simulink model "IEEE68_BUS"  (R2019b)
settings: Solver=ode15s  StartTime=0.0  StopTime=10.0  FixedStep=Ts  RelTol=1e-3
PreLoadFcn:
  | Ts=50e-5;
  | 
  | % Required data to 68 Bus benchmark
  | % clear
  | % clc
  | % Definition for the columns
  | % system base =100 MVA
  | 
  | %% Line data Format (line)
  | % All values are given on the same system base MVA
  | % 1: From bus
  | % 2: To bus
  | % 3: Resistance (pu)
  | % 4: Reactance  (pu)
  | % 5: Charge     (pu)
  | % 6: Transformer Tap Amplitute
  | % 7: base MVA
  | % 8: Nomonal Voltage (KV)
  | 
  | %1   2    3        4       5       6        7      8
  | line=[...
  | 1	54	0	     0.0181	  0	      1.025     100    138
  | 2	58	0	     0.025	  0	      1.070     100    138
  | 3	62	0	     0.02	  0	      1.070     100    138
  | 4	19	0.0007	 0.0142	  0	      1.070     100    138
  | 5	20	0.0009	 0.018	  0	      1.009     100    138
  | 6	22	0	     0.0143	  0	      1.025     100    138
  | 7	23	0.0005	 0.0272	  0	      0         100    138
  | 8	25	0.0006	 0.0232	  0	      1.025     100    138
  | 9	29	0.0008	 0.0156   0	      1.025     100    138
  | 10	31	0	     0.026	  0	      1.04      100    138
  | 11	32	0	     0.013	  0	      1.04      100    138
  | 12	36	0	     0.0075	  0	      1.04      100    138
  | 13	17	0	     0.0033	  0	      1.04      100    138
  | 14	41	0	     0.0015	  0	      1         100    138
  | 15	42	0	     0.0015	  0	      1         100    138
  | 16	18	0	     0.003	  0	      1         100    138
  | 17	36	0.0005	 0.0045	  0.32	  0         100    138
  | 17	43	0.0005	 0.0276	  0	      0         100    138
  | 18	42	0.004	 0.06	  2.25    0         100    138
  | 18	49	0.0076	 0.1141	  1.16    0	        100    138
  | 18	50	0.0012	 0.0288	  2.06	  0         100    138
  | 20	19	0.0007	 0.0138	  0       1.06	    100    138
  | 19	68	0.0016	 0.0195	  0.304	  0         100    138
  | 21	22	0.0008	 0.014	  0.2565  0	        100    138
  | 21	68	0.0008	 0.0135	  0.2548  0	        100    138
  | 22	23	0.0006	 0.0096	  0.1846  0	        100    138
  | 23	24	0.0022	 0.035	  0.361	  0         100    138
  | 24	68	0.0003	 0.0059	  0.068	  0         100    138
  | 25	26	0.0032	 0.0323	  0.531	  0         100    138
  | 25	54	0.007	 0.0086	  0.146	  0         100    138
  | 26	27	0.0014	 0.0147	  0.2396  0	        100    138
  | 26	28	0.0043	 0.0474	  0.7802  0	        100    138
  | 26	29	0.0057	 0.0625	  1.029	  0         100    138
  | 27	37	0.0013	 0.0173	  0.3216  0	        100    138
  | 27	53	0.032	 0.32	  0.41	  0         100    138
  | 29	28	0.0014	 0.0151	  0.249	  0         100    138
  | 30	31	0.0013	 0.0187	  0.333	  0         100    138
  | 30	32	0.0024	 0.0288	  0.488	  0         100    138
  | 30	53	0.0008	 0.0074	  0.48	  0         100    138
  | 30	61	0.00095	 0.00915  0.58	  0         100    138
  | 31	38	0.0011	 0.0147	  0.247	  0         100    138
  | 31	53	0.0016	 0.0163	  0.25	  0         100    138
  | 32	33	0.0008	 0.0099	  0.168	  0         100    138
  | 33	34	0.0011	 0.0157	  0.202	  0         100    138
  | 33	38	0.0036	 0.0444	  0.693	  0         100    138
  | 34	35	0.0001	 0.0074	  0	      0.946     100    138
  | 34	36	0.0033	 0.0111	  1.45	  0         100    138
  | 35	45	0.0007	 0.0175	  1.39	  0         100    138
  | 36	61	0.0011	 0.0098	  0.68	  0         100    138
  | 37	52	0.0007	 0.0082	  0.1319  0	        100    138
  | 37	68	0.0007	 0.0089	  0.1342  0	        100    138
  | 38	46	0.0022	 0.0284	  0.43	  0         100    138
  | 39	44	0	     0.0411	  0	      0         100    138
  | 39	45	0	     0.0839	  0	      0         100    138
  | 40	41	0.006	 0.084	  3.15	  0         100    138
  | 40	48	0.002	 0.022	  1.28	  0         100    138
  | 41	42	0.004	 0.06	  2.25	  0         100    138
  | 43	44	0.0001	 0.0011	  0	      0         100    138
  | 44	45	0.0025	 0.073	  0	      0         100    138
  | 45	51	0.0004	 0.0105	  0.72	  0         100    138
  | 46	49	0.0018	 0.0274	  0.27	  0         100    138
  | 47	48	0.00125	 0.0134	  0.8	  0         100    138
  | 47	53	0.0013	 0.0188	  1.31	  0         100    138
  | 50	51	0.0009	 0.0221	  1.62	  0         100    138
  | 52	55	0.0011	 0.0133	  0.2138  0	        100    138
  | 53	54	0.0035	 0.0411	  0.6987  0	        100    138
  | 54	55	0.0013	 0.0151	  0.2572  0	        100    138
  | 55	56	0.0013	 0.0213	  0.2214  0	        100    138
  | 56	57	0.0008	 0.0128	  0.1342  0	        100    138
  | 56	66	0.0008	 0.0129	  0.1382  0	        100    138
  | 57	58	0.0002	 0.0026	  0.0434  0	        100    138
  | 57	60	0.0008	 0.0112	  0.1476  0	        100    138
  | 58	59	0.0006	 0.0092	  0.113	  0         100    138
  | 58	63	0.0007	 0.0082	  0.1389  0	        100    138
  | 59	60	0.0004	 0.0046	  0.078	  0         100    138
  | 60	61	0.0023	 0.0363	  0.3804  0	        100    138
  | 62	63	0.0004	 0.0043	  0.0729  0	        100    138
  | 62	65	0.0004	 0.0043	  0.0729  0	        100    138
  | 63	64	0.0016	 0.0435	  0	      1.06      100    138
  | 65	64	0.0016	 0.0435	  0	      1.06      100    138
  | 65	66	0.0009	 0.0101	  0.1723  0 	    100    138
  | 66	67	0.0018	 0.0217	  0.366	  0         100    138
  | 67	68	0.0009	 0.0094   0.171   0         100   138 ];
  | 
  | mac_con=[
  |   1  1  200.0 0.30 0.0010  0.200 0.060 0.01  7.000 0.003 0.190 0.080 0.03  0.700 0.005 50.00 0.000 0.00 39 ;
  |   2  2  200.0 0.350 0.0270  2.950 0.697 0.01  6.560 0.003 2.820 1.7   0.03  1.500 0.005 3.030 0.000 0.00 31 ;
  |   3  3  200.0 0.304 .00386  2.495 0.531 0.01  5.700 0.003 2.370 0.876 0.03  1.500 0.005 3.580 0.000 0.00 32 ;
  |   4  4  200.0 0.295 .00222  2.620 0.436 0.01  5.690 0.003 2.580 1.66  0.03  1.500 0.005 2.860 0.000 0.00 33 ;
  |   5  5  200.0 0.540 0.0014  6.700 1.320 0.01  5.400 0.003 6.200 1.66  0.03  0.440 0.005 2.600 0.000 0.00 34 ;
  |   6  6  200.0 0.224 0.0615  2.540 0.500 0.01  7.300 0.003 2.410 0.814 0.03  0.400 0.005 3.480 0.000 0.00 35 ;
  |   7  7  200.0 0.322 .00268  2.950 0.490 0.01  5.660 0.003 2.920 1.86  0.03  1.500 0.005 2.640 0.000 0.00 36 ;
  |   8  8  200.0 0.280 .00686  2.900 0.570 0.01  6.700 0.003 2.800 0.911 0.03  0.410 0.005 2.430 0.000 0.00 37 ;
  |   9  9  200.0 0.298 0.0030  2.106 0.570 0.01  4.790 0.003 2.050 0.587 0.03  1.960 0.005 3.450 0.000 0.00 38 ;
  |   10 10 200.0 0.125 0.0014  1.000 0.310 0.01  10.20 0.003 0.690 0.08  0.03  1.500 0.005 4.200 0.000 0.00 30 ;
  |   11 11 200.0 0.125 0.0014  1.000 0.310 0.01  10.20 0.003 0.690 0.08  0.03  1.500 0.005 4.200 0.000 0.00 30 ;
  |   12 12 200.0 0.125 0.0014  1.000 0.310 0.01  10.20 0.003 0.690 0.08  0.03  1.500 0.005 4.200 0.000 0.00 30 ;
  |   13 13 6000.0 0.125 0.0014  1.000 0.310 0.01  10.20 0.003 0.690 0.08  0.03  1.500 0.005 4.200 0.000 0.00 30 ;
  |   14 14 3000.0 0.125 0.0014  1.000 0.310 0.01  10.20 0.003 0.690 0.08  0.03  1.500 0.005 4.200 0.000 0.00 30 ;
  |   15 15 3000.0 0.125 0.0014  1.000 0.310 0.01  10.20 0.003 0.690 0.08  0.03  1.500 0.005 4.200 0.000 0.00 30 ;
  |   16 16 6000.0 0.125 0.0014  1.000 0.310 0.01  10.20 0.003 0.690 0.08  0.03  1.500 0.005 4.200 0.000 0.00 30 ;];
  |   mac_con(:,5)=0;
  | 
  | p0=[250/200 545/200 650/200 632/200 505/200 700/200 560/200 540/200 800/200 500/200 1000/200 1350/200 3591/6000 1785/3000 1000/3000 3379.57/6000]%'./1000;%Active Power Generation of PV units
  | Pn(1:16,1)=1; % Nominal Power
  | 
  | 
  | %% Power System Stabilizer Format (MB)
  | % Applied power system stabilizer is MBPSS with simplified settings
  | % Note: All machines use MBPSS with same configuration
  | % 1: Global gain (G)
  | % 2: Frequency of low frequency band (FL) Hz
  | % 3: Gain of low frequency band (KL)
  | % 4: Frequency of intermediate frequency band (FI) Hz
  | % 5: Gain of intermediate frequency band (KI)
  | % 6: Frequency of high frequency band (FH) Hz
  | % 7: Gain of high frequency band (KH)
  | %   1    2  3     4   5      6  7
  | MB=[1   0.2 30   1.25 40    12 160];
  | 
  | %% Excitation System format (AVR_Data)
  | % All machines use IEEE type 1 synchronous machine voltage regulator combined to an exciter
  | % 1. Low pass filter time constant (Tr) sec
  | % 2. Regulator gain (Ka)
  | % 3. regulator time constant (Ta) sec
  | % 4. Lead-lag compensator time constant (Tb) sec
  | % 5. Lead-lag compensator time constant (Tc) sec
  | % 6. Terminal voltage (pu)
  | % 7. Lower limit for regulator output (Emin)
  | % 8. Upper limit for regulator output (Emax)
  | %     1    2      3      4     5     6       7    8
  |   AVR_Data=[...
  |     0.01  200    0.015   10    1    1.03    -5    5
  |     0.01  200    0.015   10    1    1.03    -5    5
  |     0.01  200    0.015   10    1    1.03    -5    5
  |     0.01  200    0.015   10    1    1.03    -5    5
  |     0.01  200    0.015   10    1    1.03    -5    5
  |     0.01  200    0.015   10    1    1.03    -5    5
  |     0.01  200    0.015   10    1    1.03    -5    5
  |     0.01  200    0.015   10    1    1.03    -5    5
  |     0.01  200    0.015   10    1    1.03    -5    5
  |     0.01  200    0.015   10    1    1.03    -5    5
  |     0.01  200    0.015   10    1    1.03    -5    5
  |     0.01  200    0.015   10    1    1.03    -5    5
  |     0.01  200    0.015   10    1    1.03    -5    5
  |     0.01  200    0.015   10    1    1.03    -5    5
  |     0.01  200    0.015   10    1    1.03    -5    5
  |     0.01  200    0.015   10    1    1.03    -5    5];
  | 
  | C0=829.7e-9;
  | L0=3.220e-3;
  | R0=1;
  | Ns=120*60/(2); %Nominal speed of synchronous machines
  | s=10;
  | % PSSModel=1;%1:No pSS //1:MB
  | %% Bus data (Bus)
  | % 1. Bus number
  | % 2. Nominal phase-phase voltage
  | %    1    2
  | Vg=138000;
  | Bus = [ ...
  | 1	138
  | 2	138
  | 3	138
  | 4	138
  | 5	138
  | 6	138
  | 7	138
  | 8	138
  | 9	138
  | 10	138
  | 11	138
  | 12	138
  | 13	138
  | 14	138
  | 15	138
  | 16	138
  | 17	138
  | 18	138
  | 19	138
  | 20	138
  | 21	138
  | 22	138
  | 23	138
  | 24	138
  | 25	138
  | 26	138
  | 27	138
  | 28	138
  | 29	138
  | 30	138
  | 31	138
  | 32	138
  | 33	138
  | 34	138
  | 35	138
  | 36	138
  | 37	138
  | 38	138
  | 39	138
  | 40	138
  | 41	138
  | 42	138
  | 43	138
  | 44	138
  | 45	138
  | 46	138
  | 47	138
  | 48	138
  | 49	138
  | 50	138
  | 51	138
  | 52	138
  | 53	138
  | 54	138
  | 55	138
  | 56	138
  | 57	138
  | 58	138
  | 59	138
  | 60	138
  | 61	138
  | 62	138
  | 63	138
  | 64	138
  | 65	138
  | 66	138
  | 67	138
  | 68	138];
  | 
  |    zbase=(line(:,8).^2)./line(:,7);
  |    line(:,3)=line(:,3).*zbase;
  |    line(:,4)=line(:,4).*zbase/(120*pi);
  |    line(:,5)=line(:,5)./zbase/(120*pi);
  | 
  | PSSMODEL=1;
  | LPSS=0;
  | WAPSS=0;
  | WAPSS2=0;
  | Ts=50e-5;
InitFcn:
  | PSSMODEL=1;
  | LPSS=0;
  | WAPSS=0;
  | WAPSS2=0;
  | Ts=50e-5;
  | 
  | 
  | 
  | 
  | 
  | 
  | % Required data to 68 Bus benchmark
  | % clear
  | % clc
  | % Definition for the columns
  | % system base =100 MVA
  | 
  | %% Line data Format (line)
  | % All values are given on the same system base MVA
  | % 1: From bus
  | % 2: To bus
  | % 3: Resistance (pu)
  | % 4: Reactance  (pu)
  | % 5: Charge     (pu)
  | % 6: Transformer Tap Amplitute
  | % 7: base MVA
  | % 8: Nomonal Voltage (KV)
  | 
  | %1   2    3        4       5       6        7      8
  | line=[...
  | 1	54	0	     0.0181	  0	      1.025     100    138
  | 2	58	0	     0.025	  0	      1.070     100    138
  | 3	62	0	     0.02	  0	      1.070     100    138
  | 4	19	0.0007	 0.0142	  0	      1.070     100    138
  | 5	20	0.0009	 0.018	  0	      1.009     100    138
  | 6	22	0	     0.0143	  0	      1.025     100    138
  | 7	23	0.0005	 0.0272	  0	      0         100    138
  | 8	25	0.0006	 0.0232	  0	      1.025     100    138
  | 9	29	0.0008	 0.0156   0	      1.025     100    138
  | 10	31	0	     0.026	  0	      1.04      100    138
  | 11	32	0	     0.013	  0	      1.04      100    138
  | 12	36	0	     0.0075	  0	      1.04      100    138
  | 13	17	0	     0.0033	  0	      1.04      100    138
  | 14	41	0	     0.0015	  0	      1         100    138
  | 15	42	0	     0.0015	  0	      1         100    138
  | 16	18	0	     0.003	  0	      1         100    138
  | 17	36	0.0005	 0.0045	  0.32	  0         100    138
  | 17	43	0.0005	 0.0276	  0	      0         100    138
  | 18	42	0.004	 0.06	  2.25    0         100    138
  | 18	49	0.0076	 0.1141	  1.16    0	        100    138
  | 18	50	0.0012	 0.0288	  2.06	  0         100    138
  | 20	19	0.0007	 0.0138	  0       1.06	    100    138
  | 19	68	0.0016	 0.0195	  0.304	  0         100    138
  | 21	22	0.0008	 0.014	  0.2565  0	        100    138
  | 21	68	0.0008	 0.0135	  0.2548  0	        100    138
  | 22	23	0.0006	 0.0096	  0.1846  0	        100    138
  | 23	24	0.0022	 0.035	  0.361	  0         100    138
  | 24	68	0.0003	 0.0059	  0.068	  0         100    138
  | 25	26	0.0032	 0.0323	  0.531	  0         100    138
  | 25	54	0.007	 0.0086	  0.146	  0         100    138
  | 26	27	0.0014	 0.0147	  0.2396  0	        100    138
  | 26	28	0.0043	 0.0474	  0.7802  0	        100    138
  | 26	29	0.0057	 0.0625	  1.029	  0         100    138
  | 27	37	0.0013	 0.0173	  0.3216  0	        100    138
  | 27	53	0.032	 0.32	  0.41	  0         100    138
  | 29	28	0.0014	 0.0151	  0.249	  0         100    138
  | 30	31	0.0013	 0.0187	  0.333	  0         100    138
  | 30	32	0.0024	 0.0288	  0.488	  0         100    138
  | 30	53	0.0008	 0.0074	  0.48	  0         100    138
  | 30	61	0.00095	 0.00915  0.58	  0         100    138
  | 31	38	0.0011	 0.0147	  0.247	  0         100    138
  | 31	53	0.0016	 0.0163	  0.25	  0         100    138
  | 32	33	0.0008	 0.0099	  0.168	  0         100    138
  | 33	34	0.0011	 0.0157	  0.202	  0         100    138
  | 33	38	0.0036	 0.0444	  0.693	  0         100    138
  | 34	35	0.0001	 0.0074	  0	      0.946     100    138
  | 34	36	0.0033	 0.0111	  1.45	  0         100    138
  | 35	45	0.0007	 0.0175	  1.39	  0         100    138
  | 36	61	0.0011	 0.0098	  0.68	  0         100    138
  | 37	52	0.0007	 0.0082	  0.1319  0	        100    138
  | 37	68	0.0007	 0.0089	  0.1342  0	        100    138
  | 38	46	0.0022	 0.0284	  0.43	  0         100    138
  | 39	44	0	     0.0411	  0	      0         100    138
  | 39	45	0	     0.0839	  0	      0         100    138
  | 40	41	0.006	 0.084	  3.15	  0         100    138
  | 40	48	0.002	 0.022	  1.28	  0         100    138
  | 41	42	0.004	 0.06	  2.25	  0         100    138
  | 43	44	0.0001	 0.0011	  0	      0         100    138
  | 44	45	0.0025	 0.073	  0	      0         100    138
  | 45	51	0.0004	 0.0105	  0.72	  0         100    138
  | 46	49	0.0018	 0.0274	  0.27	  0         100    138
  | 47	48	0.00125	 0.0134	  0.8	  0         100    138
  | 47	53	0.0013	 0.0188	  1.31	  0         100    138
  | 50	51	0.0009	 0.0221	  1.62	  0         100    138
  | 52	55	0.0011	 0.0133	  0.2138  0	        100    138
  | 53	54	0.0035	 0.0411	  0.6987  0	        100    138
  | 54	55	0.0013	 0.0151	  0.2572  0	        100    138
  | 55	56	0.0013	 0.0213	  0.2214  0	        100    138
  | 56	57	0.0008	 0.0128	  0.1342  0	        100    138
  | 56	66	0.0008	 0.0129	  0.1382  0	        100    138
  | 57	58	0.0002	 0.0026	  0.0434  0	        100    138
  | 57	60	0.0008	 0.0112	  0.1476  0	        100    138
  | 58	59	0.0006	 0.0092	  0.113	  0         100    138
  | 58	63	0.0007	 0.0082	  0.1389  0	        100    138
  | 59	60	0.0004	 0.0046	  0.078	  0         100    138
  | 60	61	0.0023	 0.0363	  0.3804  0	        100    138
  | 62	63	0.0004	 0.0043	  0.0729  0	        100    138
  | 62	65	0.0004	 0.0043	  0.0729  0	        100    138
  | 63	64	0.0016	 0.0435	  0	      1.06      100    138
  | 65	64	0.0016	 0.0435	  0	      1.06      100    138
  | 65	66	0.0009	 0.0101	  0.1723  0 	    100    138
  | 66	67	0.0018	 0.0217	  0.366	  0         100    138
  | 67	68	0.0009	 0.0094   0.171   0         100   138 ];
  | 
  | 
  | 
  | %% Power System Stabilizer Format (MB)
  | % Applied power system stabilizer is MBPSS with simplified settings
  | % Note: All machines use MBPSS with same configuration
  | % 1: Global gain (G)
  | % 2: Frequency of low frequency band (FL) Hz
  | % 3: Gain of low frequency band (KL)
  | % 4: Frequency of intermediate frequency band (FI) Hz
  | % 5: Gain of intermediate frequency band (KI)
  | % 6: Frequency of high frequency band (FH) Hz
  | % 7: Gain of high frequency band (KH)
  | %   1    2  3     4   5      6  7
  | MB=[1   0.2 30   1.25 40    12 160];
  | 
  | %% Excitation System format (AVR_Data)
  | % All machines use IEEE type 1 synchronous machine voltage regulator combined to an exciter
  | % 1. Low pass filter time constant (Tr) sec
  | % 2. Regulator gain (Ka)
  | % 3. regulator time constant (Ta) sec
  | % 4. Lead-lag compensator time constant (Tb) sec
  | % 5. Lead-lag compensator time constant (Tc) sec
  | % 6. Terminal voltage (pu)
  | % 7. Lower limit for regulator output (Emin)
  | % 8. Upper limit for regulator output (Emax)
  | %     1    2      3      4     5     6       7    8
  |   AVR_Data=[...
  |     0.01  200    0.015   10    1    1.03    -5    5
  |     0.01  200    0.015   10    1    1.03    -5    5
  |     0.01  200    0.015   10    1    1.03    -5    5
  |     0.01  200    0.015   10    1    1.03    -5    5
  |     0.01  200    0.015   10    1    1.03    -5    5
  |     0.01  200    0.015   10    1    1.03    -5    5
  |     0.01  200    0.015   10    1    1.03    -5    5
  |     0.01  200    0.015   10    1    1.03    -5    5
  |     0.01  200    0.015   10    1    1.03    -5    5
  |     0.01  200    0.015   10    1    1.03    -5    5
  |     0.01  200    0.015   10    1    1.03    -5    5
  |     0.01  200    0.015   10    1    1.03    -5    5
  |     0.01  200    0.015   10    1    1.03    -5    5
  |     0.01  200    0.015   10    1    1.03    -5    5
  |     0.01  200    0.015   10    1    1.03    -5    5
  |     0.01  200    0.015   10    1    1.03    -5    5];
  | 
  | C0=829.7e-9;
  | L0=3.220e-3;
  | R0=1;
  | Ns=120*60/(2); %Nominal speed of synchronous machines
  | s=10;
  | % PSSModel=1;%1:No pSS //1:MB
  | %% Bus data (Bus)
  | % 1. Bus number
  | % 2. Nominal phase-phase voltage
  | %    1    2
  | Vg=138000;
  | Bus = [ ...
  | 1	138
  | 2	138
  | 3	138
  | 4	138
  | 5	138
  | 6	138
  | 7	138
  | 8	138
  | 9	138
  | 10	138
  | 11	138
  | 12	138
  | 13	138
  | 14	138
  | 15	138
  | 16	138
  | 17	138
  | 18	138
  | 19	138
  | 20	138
  | 21	138
  | 22	138
  | 23	138
  | 24	138
  | 25	138
  | 26	138
  | 27	138
  | 28	138
  | 29	138
  | 30	138
  | 31	138
  | 32	138
  | 33	138
  | 34	138
  | 35	138
  | 36	138
  | 37	138
  | 38	138
  | 39	138
  | 40	138
  | 41	138
  | 42	138
  | 43	138
  | 44	138
  | 45	138
  | 46	138
  | 47	138
  | 48	138
  | 49	138
  | 50	138
  | 51	138
  | 52	138
  | 53	138
  | 54	138
  | 55	138
  | 56	138
  | 57	138
  | 58	138
  | 59	138
  | 60	138
  | 61	138
  | 62	138
  | 63	138
  | 64	138
  | 65	138
  | 66	138
  | 67	138
  | 68	138];
  | 
  |    zbase=(line(:,8).^2)./line(:,7);
  |    line(:,3)=line(:,3).*zbase;
  |    line(:,4)=line(:,4).*zbase/(120*pi);
  |    line(:,5)=line(:,5)./zbase/(120*pi);
  | 
  | PSSMODEL=1;
undefined symbols (not defined in the file or in its folder): D1, Delta
libraries: powerlib x359, sps_avr x16, powerlib_meascontrol x5
(part 1 of 8)
settings Model: Creator=rubai  LastModifiedBy=shamim

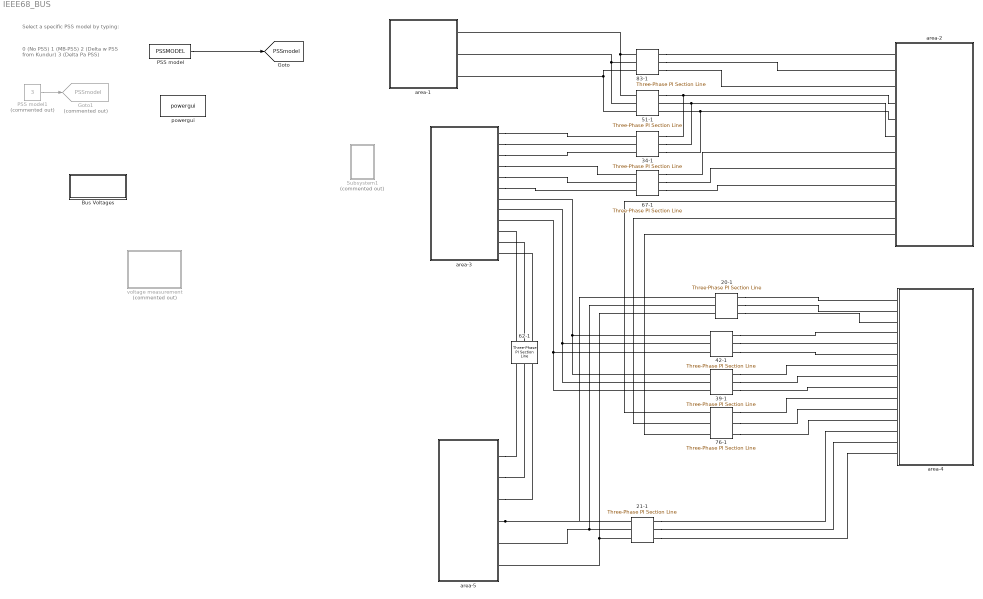
== system IEEE68_BUS ==
  note: Select a specific PSS model
      | by typing:
  note: 0  (No PSS)
      | 1  (MB-PSS)
      | 2  (Delta w PSS from Kundur)
      | 3  (Delta Pa PSS)
  20-1 : powerlib/Elements/Three-Phase PI Section Line  LConnTagsString=a|b|c  RConnTagsString=A|B|C  Frequency=60  Resistances=[line(20,3) 3*line(20,3)]  Inductances=[line(20,4) 3*line(20,4)]  Capacitances=[line(20,5) line(20,5)/3]  Length=1
      settings: SourceProductName=Simscape Electrical
  21-1 : powerlib/Elements/Three-Phase PI Section Line  LConnTagsString=a|b|c  RConnTagsString=A|B|C  Frequency=60  Resistances=[line(21,3) 3*line(21,3)]  Inductances=[line(21,4) 3*line(21,4)]  Capacitances=[line(21,5) line(21,5)/3]  Length=1
      settings: SourceProductName=Simscape Electrical
  34-1 : powerlib/Elements/Three-Phase PI Section Line  LConnTagsString=a|b|c  RConnTagsString=A|B|C  Frequency=60  Resistances=[line(34,3) 3*line(34,3)]  Inductances=[line(34,4) 3*line(34,4)]  Capacitances=[line(34,5) line(34,5)/3]  Length=1
      settings: SourceProductName=Simscape Electrical
  39-1 : powerlib/Elements/Three-Phase PI Section Line  LConnTagsString=a|b|c  RConnTagsString=A|B|C  Frequency=60  Resistances=[line(39,3) 3*line(39,3)]  Inductances=[line(39,4) 3*line(39,4)]  Capacitances=[line(39,5) line(39,5)/3]  Length=1
      settings: SourceProductName=Simscape Electrical
  42-1 : powerlib/Elements/Three-Phase PI Section Line  LConnTagsString=a|b|c  RConnTagsString=A|B|C  Frequency=60  Resistances=[line(42,3) 3*line(42,3)]  Inductances=[line(42,4) 3*line(42,4)]  Capacitances=[line(42,5) line(42,5)/3]  Length=1
      settings: SourceProductName=Simscape Electrical
  51-1 : powerlib/Elements/Three-Phase PI Section Line  LConnTagsString=a|b|c  RConnTagsString=A|B|C  Frequency=60  Resistances=[line(51,3) 3*line(51,3)]  Inductances=[line(51,4) 3*line(51,4)]  Capacitances=[line(51,5) line(51,5)/3]  Length=1
      settings: SourceProductName=Simscape Electrical
  62-1 : powerlib/Elements/Three-Phase PI Section Line  LConnTagsString=a|b|c  RConnTagsString=A|B|C  Frequency=60  Resistances=[line(62,3) 3*line(62,3)]  Inductances=[line(62,4) 3*line(62,4)]  Capacitances=[line(62,5) line(62,5)/3]  Length=1
      settings: SourceProductName=Simscape Electrical
  67-1 : powerlib/Elements/Three-Phase PI Section Line  LConnTagsString=a|b|c  RConnTagsString=A|B|C  Frequency=60  Resistances=[line(67,3) 3*line(67,3)]  Inductances=[line(67,4) 3*line(67,4)]  Capacitances="[line(67,5)  line(67,5)/3]"  Length=1
      settings: SourceProductName=Simscape Electrical
  76-1 : powerlib/Elements/Three-Phase PI Section Line  LConnTagsString=a|b|c  RConnTagsString=A|B|C  Frequency=60  Resistances=[line(76,3) 3*line(76,3)]  Inductances=[line(76,4) 3*line(76,4)]  Capacitances=[line(76,5) line(76,5)/3]  Length=1
      settings: SourceProductName=Simscape Electrical
  83-1 : powerlib/Elements/Three-Phase PI Section Line  LConnTagsString=a|b|c  RConnTagsString=A|B|C  Frequency=60  Resistances=[line(83,3) 3*line(83,3)]  Inductances=[line(83,4) 3*line(83,4)]  Capacitances=[line(83,5) line(83,5)/3]  Length=1
      settings: SourceProductName=Simscape Electrical
  "Bus Voltages " : Subsystem
  Goto1 : Goto  Commented=on  GotoTag=PSSmodel  TagVisibility=global
  PSS model : Constant  Value=PSSMODEL
  PSS model1 : Constant  Commented=on  Value=3
  Subsystem1 : Subsystem  Commented=on
  area-1 : Subsystem
  area-2 : Subsystem
  area-3 : Subsystem
  area-4 : Subsystem
  area-5 : Subsystem
  powergui : powerlib/powergui  Priority=1  SimulationMode=Phasor  SampleTime=Ts  frequency=60  Iterations=50  frequencyindice=60  Pbase=100e6  ErrMax=1e-4  UnitsV=kV  UnitsW=MW  buscounter=0  FunctionMessages=off  echomessages=off  EnableUseOfTLC=off  CurrentSourceSwitches=off  DisableSnubberDevices=off  DisableRonSwitches=off  DisableVfSwitches=off  DisplayEquations=off  AutomaticDiscreteSolvers=on  SolverType=Tustin/Backward Euler (TBE)  Interpol=off  ExternalGateDelay=off  methode=off  Ts=100  x0status=blocks  SPID=on  SwTol=0  HookPort=off  NonlinearTolerance=1e-4  nMaxIteration=100  ContinueOnMaxIteration=off  RestoreLinks=warning  ResistiveCurrentMeasurement=off  Frange=[0:2:500]  Ylog=off  Xlog=on  ShowGrid=off  save=off  variable=ZData  structure=0  ZoomFFT=off  StartTime=0.0  cycles=1  DisplayStyle=1  fundamental=60  FreqAxis=off  MaxFrequency=1000  frequencyindicesteady=1  RmsSteady=1  display=off
      settings: SourceProductName=Simscape Electrical
  "voltage measurement " : Subsystem  Commented=on
  tag scope: PSSmodel=global
  wires:
  PSS model/1 -> [PSSmodel]
  PSS model1/1 -> Goto1/1
  connections:
  83-1/RConn1 -- area-2/RConn1
  83-1/RConn2 -- area-2/RConn2
  83-1/RConn3 -- area-2/RConn3
  83-1/LConn1 -- 51-1/LConn1 -- area-1/RConn1
  83-1/LConn2 -- 51-1/LConn2 -- area-1/RConn2
  83-1/LConn3 -- 51-1/LConn3 -- area-1/RConn3
  51-1/RConn1 -- 34-1/RConn1 -- area-2/RConn4
  34-1/RConn2 -- 51-1/RConn2 -- area-2/RConn6
  34-1/RConn3 -- 51-1/RConn3 -- area-2/RConn5
  area-3/RConn1 -- 34-1/LConn1
  area-3/RConn2 -- 34-1/LConn2
  area-3/RConn3 -- 34-1/LConn3
  area-3/RConn4 -- 67-1/LConn1
  area-3/RConn5 -- 67-1/LConn2
  area-3/RConn6 -- 67-1/LConn3
  67-1/RConn1 -- area-2/RConn7
  67-1/RConn2 -- area-2/RConn8
  67-1/RConn3 -- area-2/RConn9
  42-1/LConn1 -- 39-1/LConn1 -- area-3/RConn7
  42-1/LConn2 -- 39-1/LConn2 -- area-3/RConn8
  42-1/LConn3 -- 39-1/LConn3 -- area-3/RConn9
  42-1/RConn1 -- area-4/RConn4
  42-1/RConn2 -- area-4/RConn5
  42-1/RConn3 -- area-4/RConn6
  76-1/RConn1 -- area-4/RConn10
  76-1/RConn2 -- area-4/RConn11
  76-1/RConn3 -- area-4/RConn12
  area-2/RConn10 -- 76-1/LConn1
  area-2/RConn11 -- 76-1/LConn2
  area-2/RConn12 -- 76-1/LConn3
  39-1/RConn1 -- area-4/RConn7
  39-1/RConn2 -- area-4/RConn8
  39-1/RConn3 -- area-4/RConn9
  62-1/LConn1 -- area-3/RConn10
  62-1/LConn2 -- area-3/RConn11
  62-1/LConn3 -- area-3/RConn12
  area-5/RConn1 -- 62-1/RConn1
  area-5/RConn2 -- 62-1/RConn2
  area-5/RConn3 -- 62-1/RConn3
  21-1/LConn1 -- area-4/RConn13
  21-1/LConn2 -- area-4/RConn14
  21-1/LConn3 -- area-4/RConn15
  area-5/RConn4 -- 20-1/RConn1 -- 21-1/RConn1
  21-1/RConn2 -- 20-1/RConn2 -- area-5/RConn5
  21-1/RConn3 -- 20-1/RConn3 -- area-5/RConn6
  20-1/LConn1 -- area-4/RConn1
  20-1/LConn2 -- area-4/RConn2
  20-1/LConn3 -- area-4/RConn3

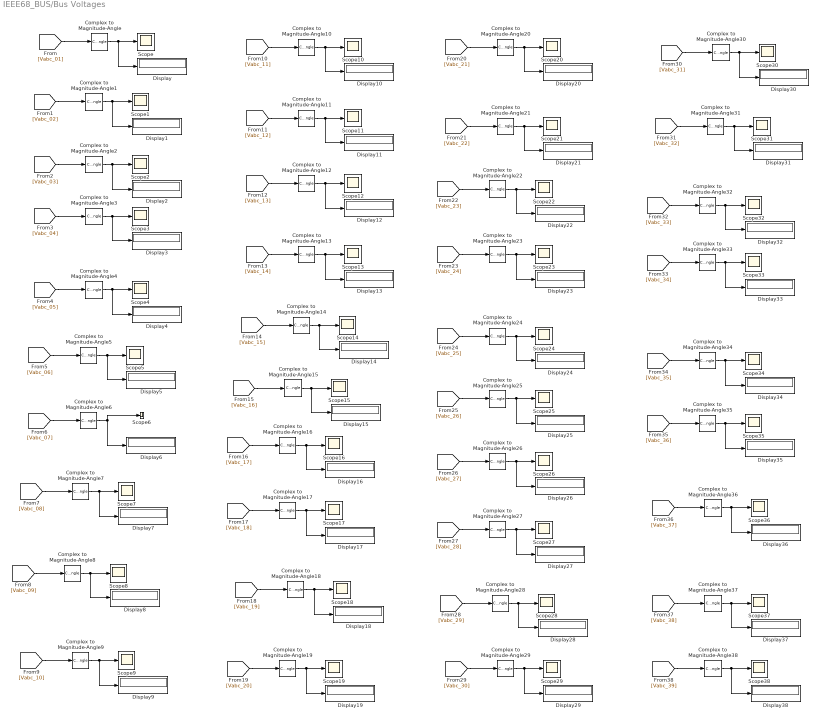
== system IEEE68_BUS/Bus Voltages  ==
  Complex to Magnitude-Angle{,1..38} (39 alike) : ComplexToMagnitudeAngle  Output=Magnitude
  Display{,1..38} (39 alike) : Display
  Scope{,1..38} (39 alike) : Scope
  wires:
  [Vabc_01] -> Complex to Magnitude-Angle/1
  Complex to Magnitude-Angle/1 -> Display/1, Scope/1
  [Vabc_02] -> Complex to Magnitude-Angle1/1
  Complex to Magnitude-Angle1/1 -> Display1/1, Scope1/1
  [Vabc_03] -> Complex to Magnitude-Angle2/1
  Complex to Magnitude-Angle2/1 -> Display2/1, Scope2/1
  [Vabc_04] -> Complex to Magnitude-Angle3/1
  Complex to Magnitude-Angle3/1 -> Display3/1, Scope3/1
  [Vabc_05] -> Complex to Magnitude-Angle4/1
  Complex to Magnitude-Angle4/1 -> Display4/1, Scope4/1
  [Vabc_06] -> Complex to Magnitude-Angle5/1
  Complex to Magnitude-Angle5/1 -> Display5/1, Scope5/1
  [Vabc_07] -> Complex to Magnitude-Angle6/1
  Complex to Magnitude-Angle6/1 -> Display6/1, Scope6/1
  [Vabc_08] -> Complex to Magnitude-Angle7/1
  Complex to Magnitude-Angle7/1 -> Display7/1, Scope7/1
  [Vabc_09] -> Complex to Magnitude-Angle8/1
  Complex to Magnitude-Angle8/1 -> Display8/1, Scope8/1
  [Vabc_10] -> Complex to Magnitude-Angle9/1
  Complex to Magnitude-Angle9/1 -> Display9/1, Scope9/1
  [Vabc_11] -> Complex to Magnitude-Angle10/1
  Complex to Magnitude-Angle10/1 -> Display10/1, Scope10/1
  [Vabc_12] -> Complex to Magnitude-Angle11/1
  Complex to Magnitude-Angle11/1 -> Display11/1, Scope11/1
  [Vabc_13] -> Complex to Magnitude-Angle12/1
  Complex to Magnitude-Angle12/1 -> Display12/1, Scope12/1
  [Vabc_14] -> Complex to Magnitude-Angle13/1
  Complex to Magnitude-Angle13/1 -> Display13/1, Scope13/1
  [Vabc_15] -> Complex to Magnitude-Angle14/1
  Complex to Magnitude-Angle14/1 -> Display14/1, Scope14/1
  Complex to Magnitude-Angle15/1 -> Scope15/1, Display15/1
  [Vabc_16] -> Complex to Magnitude-Angle15/1
  [Vabc_17] -> Complex to Magnitude-Angle16/1
  Complex to Magnitude-Angle16/1 -> Display16/1, Scope16/1
  Complex to Magnitude-Angle17/1 -> Scope17/1, Display17/1
  [Vabc_18] -> Complex to Magnitude-Angle17/1
  [Vabc_19] -> Complex to Magnitude-Angle18/1
  Complex to Magnitude-Angle18/1 -> Display18/1, Scope18/1
  Complex to Magnitude-Angle19/1 -> Scope19/1, Display19/1
  [Vabc_20] -> Complex to Magnitude-Angle19/1
  Complex to Magnitude-Angle20/1 -> Scope20/1, Display20/1
  [Vabc_21] -> Complex to Magnitude-Angle20/1
  [Vabc_22] -> Complex to Magnitude-Angle21/1
  Complex to Magnitude-Angle21/1 -> Display21/1, Scope21/1
  Complex to Magnitude-Angle22/1 -> Scope22/1, Display22/1
  [Vabc_23] -> Complex to Magnitude-Angle22/1
  [Vabc_24] -> Complex to Magnitude-Angle23/1
  Complex to Magnitude-Angle23/1 -> Display23/1, Scope23/1
  Complex to Magnitude-Angle24/1 -> Scope24/1, Display24/1
  [Vabc_25] -> Complex to Magnitude-Angle24/1
  [Vabc_26] -> Complex to Magnitude-Angle25/1
  Complex to Magnitude-Angle25/1 -> Display25/1, Scope25/1
  Complex to Magnitude-Angle26/1 -> Scope26/1, Display26/1
  [Vabc_27] -> Complex to Magnitude-Angle26/1
  [Vabc_28] -> Complex to Magnitude-Angle27/1
  Complex to Magnitude-Angle27/1 -> Display27/1, Scope27/1
  Complex to Magnitude-Angle28/1 -> Scope28/1, Display28/1
  [Vabc_29] -> Complex to Magnitude-Angle28/1
  [Vabc_30] -> Complex to Magnitude-Angle29/1
  Complex to Magnitude-Angle29/1 -> Display29/1, Scope29/1
  Complex to Magnitude-Angle30/1 -> Scope30/1, Display30/1
  [Vabc_31] -> Complex to Magnitude-Angle30/1
  [Vabc_32] -> Complex to Magnitude-Angle31/1
  Complex to Magnitude-Angle31/1 -> Display31/1, Scope31/1
  Complex to Magnitude-Angle32/1 -> Scope32/1, Display32/1
  [Vabc_33] -> Complex to Magnitude-Angle32/1
  [Vabc_34] -> Complex to Magnitude-Angle33/1
  Complex to Magnitude-Angle33/1 -> Display33/1, Scope33/1
  Complex to Magnitude-Angle34/1 -> Scope34/1, Display34/1
  [Vabc_35] -> Complex to Magnitude-Angle34/1
  [Vabc_36] -> Complex to Magnitude-Angle35/1
  Complex to Magnitude-Angle35/1 -> Display35/1, Scope35/1
  Complex to Magnitude-Angle36/1 -> Scope36/1, Display36/1
  [Vabc_37] -> Complex to Magnitude-Angle36/1
  [Vabc_38] -> Complex to Magnitude-Angle37/1
  Complex to Magnitude-Angle37/1 -> Display37/1, Scope37/1
  Complex to Magnitude-Angle38/1 -> Scope38/1, Display38/1
  [Vabc_39] -> Complex to Magnitude-Angle38/1

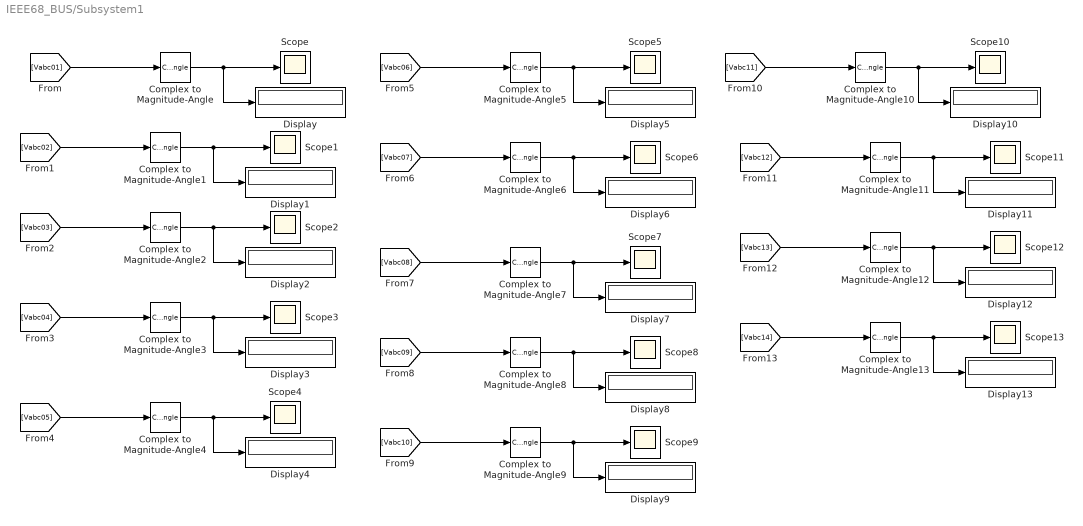
== system IEEE68_BUS/Subsystem1 ==
  Complex to Magnitude-Angle{,1..13} (14 alike) : ComplexToMagnitudeAngle  Output=Magnitude
  Display{,1..13} (14 alike) : Display
  Scope{,1..13} (14 alike) : Scope
  wires:
  Complex to Magnitude-Angle/1 -> Display/1, Scope/1
  [Vabc01] -> Complex to Magnitude-Angle/1
  [Vabc02] -> Complex to Magnitude-Angle1/1
  Complex to Magnitude-Angle1/1 -> Display1/1, Scope1/1
  [Vabc03] -> Complex to Magnitude-Angle2/1
  Complex to Magnitude-Angle2/1 -> Display2/1, Scope2/1
  [Vabc04] -> Complex to Magnitude-Angle3/1
  Complex to Magnitude-Angle3/1 -> Display3/1, Scope3/1
  [Vabc05] -> Complex to Magnitude-Angle4/1
  Complex to Magnitude-Angle4/1 -> Display4/1, Scope4/1
  [Vabc06] -> Complex to Magnitude-Angle5/1
  Complex to Magnitude-Angle5/1 -> Display5/1, Scope5/1
  [Vabc07] -> Complex to Magnitude-Angle6/1
  Complex to Magnitude-Angle6/1 -> Display6/1, Scope6/1
  [Vabc08] -> Complex to Magnitude-Angle7/1
  Complex to Magnitude-Angle7/1 -> Display7/1, Scope7/1
  [Vabc09] -> Complex to Magnitude-Angle8/1
  Complex to Magnitude-Angle8/1 -> Display8/1, Scope8/1
  [Vabc10] -> Complex to Magnitude-Angle9/1
  Complex to Magnitude-Angle9/1 -> Display9/1, Scope9/1
  [Vabc11] -> Complex to Magnitude-Angle10/1
  Complex to Magnitude-Angle10/1 -> Display10/1, Scope10/1
  [Vabc12] -> Complex to Magnitude-Angle11/1
  Complex to Magnitude-Angle11/1 -> Display11/1, Scope11/1
  [Vabc13] -> Complex to Magnitude-Angle12/1
  Complex to Magnitude-Angle12/1 -> Display12/1, Scope12/1
  [Vabc14] -> Complex to Magnitude-Angle13/1
  Complex to Magnitude-Angle13/1 -> Display13/1, Scope13/1
